simulink model "prob_19"  (R2015a)
settings: Solver=ode45  StartTime=0.0  StopTime=50  RelTol=1e-3
settings Model: Creator=Anu  LastModifiedBy=Anu

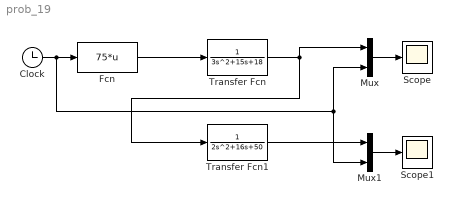
== system prob_19 ==
  Clock : Clock
  Fcn : Fcn  Expr=75*u
  Mux : Mux  Inputs=2
  Mux1 : Mux  Inputs=2
  Scope : Scope
  Scope1 : Scope
  Transfer Fcn : TransferFcn  Denominator=[3 15 18]
  Transfer Fcn1 : TransferFcn  Denominator=[2 16 50]
  wires:
  Clock/1 -> Mux/2, Mux1/2, Fcn/1
  Fcn/1 -> Transfer Fcn/1
  Transfer Fcn/1 -> Mux/1, Transfer Fcn1/1
  Mux1/1 -> Scope1/1
  Mux/1 -> Scope/1
  Transfer Fcn1/1 -> Mux1/1
